simulink model "S12_PTR_Renderer_Core_v10"  (R2026a)
settings: Solver=FixedStepDiscrete  StopTime=89.98  FixedStep=0.02
settings Model: Creator=Jovi  LastModifiedBy=Jovi

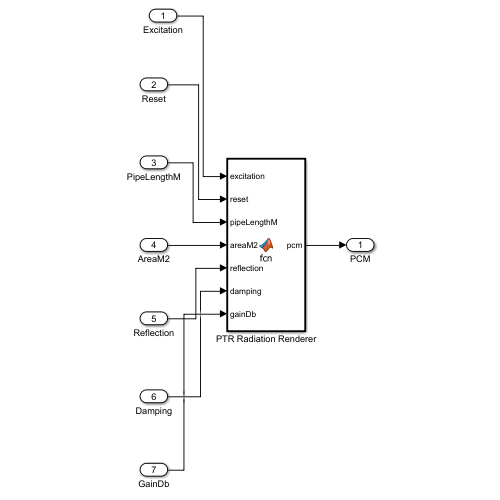
[thumbnail: Simulink's stored preview of the top-level diagram]
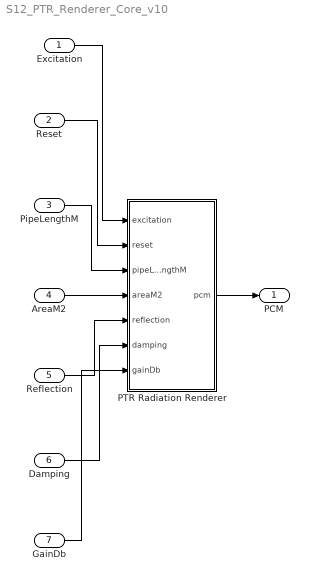
== system S12_PTR_Renderer_Core_v10 ==
  Excitation : Inport  OutDataTypeStr=double  PortDimensions=[960 1]
  Reset : Inport  Port=2  OutDataTypeStr=boolean  PortDimensions=1
  PipeLengthM : Inport  Port=3  OutDataTypeStr=double  PortDimensions=1
  AreaM2 : Inport  Port=4  OutDataTypeStr=double  PortDimensions=1
  Reflection : Inport  Port=5  OutDataTypeStr=double  PortDimensions=1
  Damping : Inport  Port=6  OutDataTypeStr=double  PortDimensions=1
  GainDb : Inport  Port=7  OutDataTypeStr=double  PortDimensions=1
  PTR Radiation Renderer : MATLAB Function  TreatAsAtomicUnit=on
  PCM : Outport  OutDataTypeStr=double  PortDimensions=[960 2]
  wires:
  Excitation/1 -> PTR Radiation Renderer/1(excitation)
  Reset/1 -> PTR Radiation Renderer/2(reset)
  PipeLengthM/1 -> PTR Radiation Renderer/3(pipeLengthM)
  AreaM2/1 -> PTR Radiation Renderer/4(areaM2)
  Reflection/1 -> PTR Radiation Renderer/5(reflection)
  Damping/1 -> PTR Radiation Renderer/6(damping)
  GainDb/1 -> PTR Radiation Renderer/7(gainDb)
  PTR Radiation Renderer/1(pcm) -> PCM/1

== matlab function S12_PTR_Renderer_Core_v10/PTR Radiation Renderer ==
  data: excitation input; pcm output; reset input; pipeLengthM input; areaM2 input; reflection input; damping input; gainDb input
function pcm = fcn(excitation, reset, pipeLengthM, areaM2, reflection, damping, gainDb)
%#codegen
pressure = s12_sound_playground_ptr_tuning_step(excitation, pipeLengthM, areaM2, reflection, damping, reset);
gain = 10^(gainDb / 20);
pcm = gain * [pressure, 0.985 * pressure];
end
